simulink model "Impulse_simulation"  (R2015b)
settings: Solver=VariableStepAuto  StartTime=0.0  StopTime=0.16  RelTol=1e-3
libraries: fl_lib x10, nesl_utility x3, elec_lib x1
settings Model: Creator=gbz  LastModifiedBy=gbz

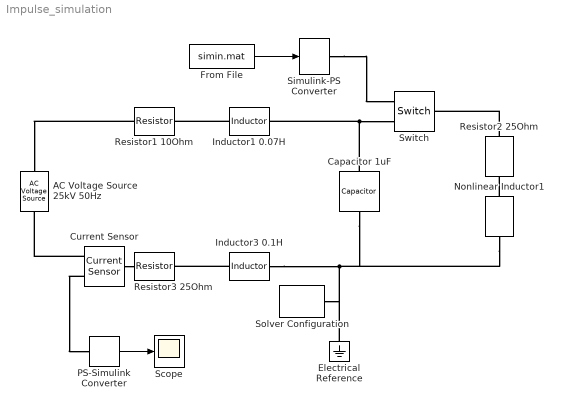
== system Impulse_simulation ==
  AC Voltage Source 25kV 50Hz : fl_lib/Electrical/Electrical Sources/AC Voltage Source  amp=25000 V  shift=0 deg  frequency=50 Hz  omega=0 rad/s
  Capacitor 1uF : fl_lib/Electrical/Electrical Elements/Capacitor  c=1 uF  r=1e-6 Ohm  g=0 1/Ohm  i_specify=off  i_priority=None  i=0 A  v_specify=off  v_priority=None  v=0 V  vc_specify=off  vc_priority=None  vc=0 V
  Current Sensor : fl_lib/Electrical/Electrical Sensors/Current Sensor
  Electrical Reference : fl_lib/Electrical/Electrical Elements/Electrical Reference
  From File : FromFile  FileName=simin.mat
  Inductor1 0.07H : fl_lib/Electrical/Electrical Elements/Inductor  l=0.07 H  r=0 Ohm  g=1e-9 1/Ohm  i_specify=off  i_priority=None  i=0 A  v_specify=off  v_priority=None  v=0 V  i_L_specify=off  i_L_priority=None  i_L=0 A
  Inductor3 0.1H : fl_lib/Electrical/Electrical Elements/Inductor  l=0.08 H  r=0 Ohm  g=1e-9 1/Ohm  i_specify=off  i_priority=None  i=0 A  v_specify=off  v_priority=None  v=0 V  i_L_specify=off  i_L_priority=None  i_L=0 A
  Nonlinear Inductor1 : elec_lib/Passive Devices/Nonlinear Inductor  parameterization_option=2  Nw=10  L=2e-4 H  L_sat=1e-4 H  current_data=[ 0 0.64 1.28 1.92 2.56 3.20 ] A  magnetic_flux_data=[0 1.29 2.00 2.27 2.36 2.39 ].*1e-5 Wb  H_data=[ 0 200 400 600 800 1000 ] A/m  B_data=[ 0 0.81 1.25 1.42 1.48 1.49 ] T  magnetic_flux_sat=1.3e-5 Wb  length_effective=0.032 m  area_effective=1.6e-5 m^2  dBdH0=0.005 m*T/A  B1=1.49 T  H1=1000 A/m  c=0.1  K=200 A/m  alpha=1e-4  x0_option=1  i_L0=0 A  phi0=0 Wb  B0=0 T  H0=0 A/m  G_parasitic=1e-9 1/Ohm  interpolation_option=1
  PS-Simulink Converter : nesl_utility/PS-Simulink Converter  PhysicalDomain=network_engine_domain  SubClassName=ps_output  LeftPortType=input  RightPortType=output  PseudoPeriodic=off  Frequencies=[]  Unit=1  AffineConversion=off
  "Resistor1 10Ohm " : fl_lib/Electrical/Electrical Elements/Resistor  R=10 Ohm  i_specify=off  i_priority=None  i=0 A  v_specify=off  v_priority=None  v=0 V
  "Resistor2 25Ohm " : fl_lib/Electrical/Electrical Elements/Resistor  R=25 Ohm  i_specify=off  i_priority=None  i=0 A  v_specify=off  v_priority=None  v=0 V
  Resistor3 25Ohm : fl_lib/Electrical/Electrical Elements/Resistor  R=25 Ohm  i_specify=off  i_priority=None  i=0 A  v_specify=off  v_priority=None  v=0 V
  Scope : Scope
  Simulink-PS Converter : nesl_utility/Simulink-PS Converter  PhysicalDomain=network_engine_domain  SubClassName=ps_input  LeftPortType=input  RightPortType=output  PseudoPeriodic=off  Frequencies=[]  NoiseDistribution=none  NoiseParameters=[]  Unit=1  AffineConversion=off  InputFiltering=off  SimscapeFilterOrder=1  InputFilterTimeConstant=0.001  UdotUserProvided=1
  Solver Configuration : nesl_utility/Solver Configuration  PhysicalDomain=network_engine_domain  SubClassName=solver  LeftPortType=input  RightPortType=generic  Accelerate=off  Tones=[]  Harmonics=[]  SimulateNoise=off  Profile=off  UseLocalSampling=off  EnableSwitchedLinearOptims=on  FrequencyDomain=off  UseCCode=off  RelTol=0.001  AbsTol=1e-06  MinStep=1e-09  ToWorkspace=off  RevertToSquareIcSolve=off  NumHomotopyIterations=100  PhasorMode=off  PhasorModeNumHarmonics=1  DoDC=off  ResidualTolerance=1e-09  UseLocalSolver=off  LocalSolverChoice=NE_BACKWARD_EULER_ADVANCER  LocalSolverSampleTime=0.001  DoFixedCost=off  MaxNonlinIter=3  MaxModeIter=2  LinearAlgebra=Sparse  DelaysMemoryBudget=1024  AutomaticFiltering=on  FilteringTimeConstant=0.001
  Switch : fl_lib/Electrical/Electrical Elements/Switch  R_closed=0.01 Ohm  G_open=1e-8 1/Ohm  Threshold=0  i_specify=off  i_priority=None  i=0 A  v_specify=off  v_priority=None  v=0 V
  wires:
  From File/1 -> Simulink-PS Converter/1
  PS-Simulink Converter/1 -> Scope/1
  connections:
  "Resistor1 10Ohm "/LConn1 -- AC Voltage Source 25kV 50Hz/LConn1
  Inductor1 0.07H/LConn1 -- "Resistor1 10Ohm "/RConn1
  Nonlinear Inductor1/LConn1 -- "Resistor2 25Ohm "/RConn1
  Inductor3 0.1H/RConn1 -- Nonlinear Inductor1/RConn1 -- Capacitor 1uF/RConn1 -- Solver Configuration/RConn1 -- Electrical Reference/LConn1
  Inductor3 0.1H/LConn1 -- Resistor3 25Ohm/RConn1
  Capacitor 1uF/LConn1 -- Switch/RConn2 -- Inductor1 0.07H/RConn1
  "Resistor2 25Ohm "/LConn1 -- Switch/LConn1
  Simulink-PS Converter/RConn1 -- Switch/RConn1
  Current Sensor/LConn1 -- Resistor3 25Ohm/LConn1
  Current Sensor/RConn2 -- AC Voltage Source 25kV 50Hz/RConn1
  Current Sensor/RConn1 -- PS-Simulink Converter/LConn1
